simulink subsystem "PieroControladoVPIZ"  (R2023b)
settings: Solver=VariableStepAuto  StartTime=0.0  StopTime=10.0  RelTol=1e-3
settings Model: Creator=Carlos  LastModifiedBy=Carlos

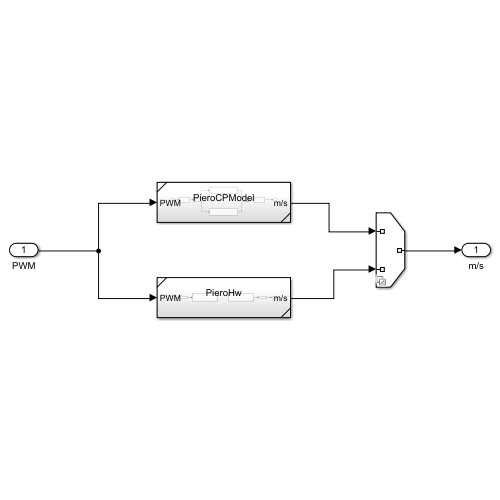
[thumbnail: Simulink's stored preview of the top-level diagram]
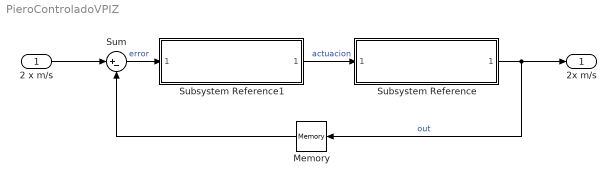
== system PieroControladoVPIZ ==
  2 x m/s : Inport
  Memory : Memory
  Subsystem Reference : Subsystem  ReferencedSubsystem=PieroCPZ
  Subsystem Reference1 : Subsystem  ReferencedSubsystem=ControladorPIZ
  Sum : Sum  Inputs=|+-
  2x m/s : Outport
  wires:
  Subsystem Reference1/1 -> Subsystem Reference/1  "actuacion"
  2 x m/s/1 -> Sum/1
  Sum/1 -> Subsystem Reference1/1  "error"
  Subsystem Reference/1 -> 2x m/s/1, Memory/1  "out"
  Memory/1 -> Sum/2
